simulink model "solution"  (R2017b)
settings: Solver=FixedStepDiscrete  StartTime=0.0  StopTime=50  FixedStep=0.01  RelTol=1e-3
settings Model: Creator=ashwin.ramanujam  LastModifiedBy=ashwin.ramanujam

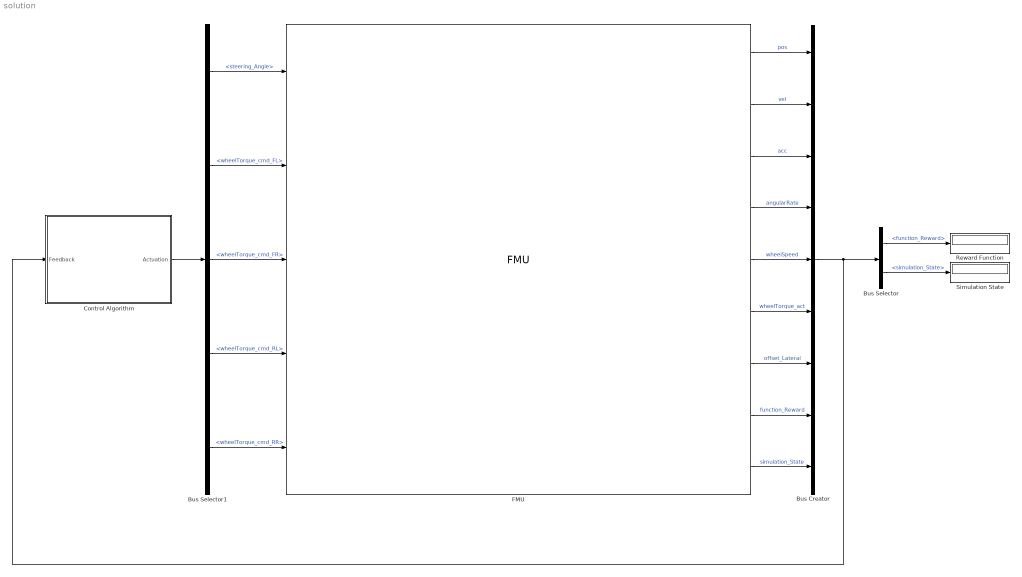
== system solution ==
  Bus Creator : BusCreator  Inputs=9
  Bus Selector : BusSelector  OutputSignals=function_Reward,simulation_State
  Bus Selector1 : BusSelector  OutputSignals=steering_Angle,wheelTorque_cmd_FL,wheelTorque_cmd_FR,wheelTorque_cmd_RL,wheelTorque_cmd_RR
  Control Algorithm : Subsystem
  FMU : FMU  FMUName=MED2018_VehicleModel.fmu  FMUDebugLogging=on  FMUMode=CoSimulation  FMUSampleTime=-1  mask(MED2018.VehicleModel [Co-Simulation, v2.0]){}
      mask Display:
      | if (exist([Simulink.fileGenControl('get','CacheFolder') '\slprj\_fmu\ee3b8d1c4fd885d6e0d545a7b9ef6a46\MED2018_VehicleModel\model.png'],'file'))
      |     image([Simulink.fileGenControl('get','CacheFolder') '\slprj\_fmu\ee3b8d1c4fd885d6e0d545a7b9ef6a46\MED2018_VehicleModel\model.png']);
      |     text(0.03, 0.97, 'MED2018.VehicleModel', 'horizontalAlignment', 'left', 'verticalAlignment', 'top');
      | else
      |     disp('MED2018.VehicleModel');
      | end
      | port_label('output',1,'Position');
      | port_label('output',2,'Velocity');
      | port_label('output',3,'Acceleration');
      | port_label('output',4,'angularRate');
      | port_label('output',5,'wheelSpeed');
      | port_label('output',6,'wheelTorque_act');
      | port_label('output',7,'offset_Lateral');
      | port_label('output',8,'function_Reward');
      | port_label('output',9,'simulation_State');
      | port_label('input',1,'steering_Angle');
      | port_label('input',2,'wheelTorque_cmd_FL');
      | port_label('input',3,'wheelTorque_cmd_FR');
      | port_label('input',4,'wheelTorque_cmd_RL');
      | port_label('input',5,'wheelTorque_cmd_RR');
  Reward Function : Display
  Simulation State : Display
  wires:
  Control Algorithm/1(Actuation) -> Bus Selector1/1
  Bus Selector1/1 -> FMU/1  "<steering_Angle>"
  Bus Selector1/2 -> FMU/2  "<wheelTorque_cmd_FL>"
  Bus Selector1/3 -> FMU/3  "<wheelTorque_cmd_FR>"
  Bus Selector1/4 -> FMU/4  "<wheelTorque_cmd_RL>"
  Bus Selector1/5 -> FMU/5  "<wheelTorque_cmd_RR>"
  Bus Creator/1 -> Bus Selector/1, Control Algorithm/1(Feedback)
  Bus Selector/1 -> Reward Function/1  "<function_Reward>"
  Bus Selector/2 -> Simulation State/1  "<simulation_State>"
  FMU/1 -> Bus Creator/1  "pos"
  FMU/2 -> Bus Creator/2  "vel"
  FMU/3 -> Bus Creator/3  "acc"
  FMU/4 -> Bus Creator/4  "angularRate"
  FMU/5 -> Bus Creator/5  "wheelSpeed"
  FMU/6 -> Bus Creator/6  "wheelTorque_act"
  FMU/7 -> Bus Creator/7  "offset_Lateral"
  FMU/8 -> Bus Creator/8  "function_Reward"
  FMU/9 -> Bus Creator/9  "simulation_State"

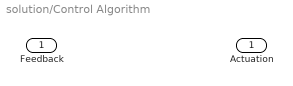
== system solution/Control Algorithm ==
  Feedback : Inport
  Actuation : Outport
